simulink model "Nexonar_Navigation"  (R2018b)
settings: Solver=FixedStepDiscrete  StartTime=0.0  StopTime=0.1  RelTol=1e-3  EnableMultiTasking=on
libraries: commutil2 x12, c2833xlib x5, c280xlib x5, simulink x1, c2000lib x1
(part 2 of 2)

== stateflow chart Nexonar_Navigation/Nexonar-System/Navigationssystem [Einstellungen moeglich]/Fahrsystem ==
  state Fahren_mit_Ausrichtungsregelung
    entry:
    pwm_out_l = pwm_out - round(pwm_mindern(1) * (pwm_out / 100) ^ 2) * l_mindern;
    pwm_out_r = pwm_out - round(pwm_mindern(1) * (pwm_out / 100) ^ 2) * r_mindern;
    r_l_out_l = 1 - Gang;
    r_l_out_r = 1 - Gang;
  state Start_Warten
  state Drehen_links_max
    entry:
    pwm_out_l = 100;
    pwm_out_r = 100;
    r_l_out_l = 0;
    r_l_out_r = 1;
  state Drehen_rechts_max
    entry:
    pwm_out_l = 100;
    pwm_out_r = 100;
    r_l_out_l = 1;
    r_l_out_r = 0;
  state Drehen_links_gesteuert
    entry:
    pwm_out_l = 59 + abs(alpha_diff_opt);
    pwm_out_r = 59 + abs(alpha_diff_opt);
    r_l_out_l = 0;
    r_l_out_r = 1;
  state Drehen_rechts_gesteuert
    entry:
    pwm_out_l = 59 + abs(alpha_diff_opt);
    pwm_out_r = 59 + abs(alpha_diff_opt);
    r_l_out_l = 1;
    r_l_out_r = 0;
  (junction 81) -> Fahren_mit_Ausrichtungsregelung [order 1] : [pwm_mindern(2) == 1]
      | {l_mindern = 1 - Gang; r_mindern = 0 + Gang;}
  (junction 81) -> Fahren_mit_Ausrichtungsregelung [order 2] : [pwm_mindern(2) == 0]
      | {l_mindern = 0 + Gang; r_mindern = 1 - Gang;}
  (junction 1) -> (junction 81) [order 2]
  Fahren_mit_Ausrichtungsregelung -> (junction 32)
  (junction 81) -> Fahren_mit_Ausrichtungsregelung [order 3] : {l_mindern = 0; r_mindern = 0;}
  Start_Warten -> (junction 1)
  (junction 32) -> (junction 1)
  (default) -> Start_Warten
  Drehen_links_max -> (junction 32)
  Drehen_rechts_max -> (junction 32)
  Drehen_links_gesteuert -> (junction 32)
  (junction 1) -> (junction 18) [order 1] : [abs(alpha_diff_opt) > 0 && pwm_out > 0]
  Drehen_rechts_gesteuert -> (junction 32)
  (junction 18) -> (junction 44) [order 1] : [abs(alpha_diff_opt) > 40]
  (junction 44) -> Drehen_links_max [order 1] : [alpha_diff_opt > 0]
  (junction 18) -> (junction 52) [order 2]
  (junction 44) -> Drehen_rechts_max [order 2]
  (junction 52) -> Drehen_links_gesteuert [order 1] : [alpha_diff_opt > 0]
  (junction 52) -> Drehen_rechts_gesteuert [order 2]
  data: Gang input; pwm_out input; pwm_mindern input; alpha_diff_opt input; pwm_out_l output; pwm_out_r output; r_l_out_l output; r_l_out_r output; l_mindern local; r_mindern local

== stateflow chart Nexonar_Navigation/Nexonar-System/Navigationssystem [Einstellungen moeglich]/Drehweg-Optimierung mit Gang-Ausrichtung [Init: Stillstandintervall = ±15°] ==
  state Einstellung_Init
    entry:
    Stillstandintervall = 15;
    %%%
    pwm_mindern = [0 0];
  state Drehstillstand_mit_Ausrichtungsregelung
    entry:
    alpha_diff_opt = 0;
    if abs(alpha_diff_intern) < 5
    pwm_mindern(1) = round(abs(alpha_diff_intern));
    elseif abs(alpha_diff_intern) < 15
    pwm_mindern(1) = 5 + floor((abs(alpha_diff_intern) - 5) / 2);
    else
    pwm_mindern(1) = 10;
    end;
    if alpha_diff_intern < 0
    pwm_mindern(2) = 0;
    elseif alpha_diff_intern > 0
    pwm_mindern(2) = 1;
    else
    pwm_mindern(2) = 2;
    end;
  state Weiterleitung_bei_Drehzustand
    entry:
    alpha_diff_opt = alpha_diff_intern;
  (default) -> Einstellung_Init
  (junction 95) -> (junction 32)
  Einstellung_Init -> (junction 32)
  (junction 32) -> (junction 6) : {alpha_diff_intern = alpha_diff + 180 * Gang}
  (junction 6) -> (junction 68) [order 2]
  (junction 68) -> Drehstillstand_mit_Ausrichtungsregelung [order 1] : [abs(alpha_diff_intern) <= Stillstandintervall]
  Drehstillstand_mit_Ausrichtungsregelung -> (junction 95)
  (junction 6) -> (junction 13) [order 1] : [abs(alpha_diff_intern) > 180]
  (junction 13) -> (junction 68) [order 1] : [alpha_diff_intern > 0]
      | {alpha_diff_intern = -360 + alpha_diff_intern}
  Weiterleitung_bei_Drehzustand -> (junction 95)
  (junction 13) -> (junction 68) [order 2] : {alpha_diff_intern = 360 + alpha_diff_intern}
  (junction 68) -> Weiterleitung_bei_Drehzustand [order 2]
  data: pwm_mindern output; Gang input; alpha_diff input; alpha_diff_opt output; alpha_diff_intern local; Stillstandintervall local

== stateflow chart Nexonar_Navigation/Nexonar-System/Navigationssystem [Einstellungen moeglich]/Winkelregelungssystem (Soll-Ist-Abgleich & Ausrichtungsauswertung)/Quadrantenteiler ==
  state Quadrant_a
    entry:
    Quadrant = 0;
  state Quadrant_b
    entry:
    Quadrant = 1;
  state Start_Warten
  state Quadrant_c
    entry:
    Quadrant = 2;
  state Quadrant_d
    entry:
    Quadrant = 3;
  (junction 6) -> Quadrant_a [order 1] : [x_diff >= 0 && y_diff >= 0]
  Quadrant_a -> (junction 35)
  (junction 6) -> Quadrant_b [order 2] : [x_diff <= 0 && y_diff > 0]
  Quadrant_b -> (junction 35)
  Start_Warten -> (junction 6)
  (junction 35) -> (junction 6)
  (default) -> Start_Warten
  (junction 6) -> Quadrant_c [order 3] : [x_diff < 0 && y_diff <= 0]
  Quadrant_c -> (junction 35)
  (junction 6) -> Quadrant_d [order 4]
  Quadrant_d -> (junction 35)
  data: x_diff input; y_diff input; Quadrant output

== stateflow chart Nexonar_Navigation/Nexonar-System/Navigationssystem [Einstellungen moeglich]/Winkelregelungssystem (Soll-Ist-Abgleich & Ausrichtungsauswertung)/Winkelausgabe fuer Ausrichtung ==
  state Ausrichtung_ohne_Aenderung
    entry:
    alpha_neu = alpha_Wagen;
  state Start_Warten
  state Trigonometrische_Auswertung_in_Grad_fuer_Quadrant_1_3
    entry:
    alpha_neu = round(atan(abs(x_diff)/abs(y_diff))*360/(2*pi));
  state Trigonometrische_Auswertung_in_Grad_fuer_Quadrant_0_2
    entry:
    alpha_neu = round(atan(abs(y_diff)/abs(x_diff))*360/(2*pi));
  (junction 4) -> Ausrichtung_ohne_Aenderung [order 1] : [x_diff == 0 && y_diff == 0]
  Ausrichtung_ohne_Aenderung -> (junction 65)
  Start_Warten -> (junction 4)
  (junction 65) -> (junction 4)
  (default) -> Start_Warten
  (junction 4) -> Trigonometrische_Auswertung_in_Grad_fuer_Quadrant_1_3 [order 4]
  (junction 4) -> Trigonometrische_Auswertung_in_Grad_fuer_Quadrant_0_2 [order 2] : [x_diff > 0 && y_diff >= 0]
  Trigonometrische_Auswertung_in_Grad_fuer_Quadrant_0_2 -> (junction 65)
  (junction 4) -> Trigonometrische_Auswertung_in_Grad_fuer_Quadrant_0_2 [order 3] : [x_diff < 0 && y_diff <= 0]
  Trigonometrische_Auswertung_in_Grad_fuer_Quadrant_1_3 -> (junction 65)
  data: x_diff input; y_diff input; alpha_neu output; alpha_Wagen input

== stateflow chart Nexonar_Navigation/Nexonar-System/Nexonar-Positionsbestimmung/Chart2 ==
  state Daten_einlesen
  state x0
  state x1_1
    entry: int16y_bin[0] = int8y_1[0];
    int16y_bin[1] = int8y_1[1];
    int16y_bin[2] = int8y_1[2];
    int16y_bin[3] = int8y_1[3];
    int16y_bin[4] = int8y_1[4];
    int16y_bin[5] = int8y_1[5]
    int16y_bin[6] = int8y_1[6];
    int16y_bin[7] = int8y_1[7];
    int16y_bin[8] = int8y_2[0];
    int16y_bin[9] = int8y_2[1];
    int16y_bin[10] = int8y_2[2];
    int16y_bin[11] = int8y_2[3];
    int16y_bin[12] = int8y_2[4];
    int16y_bin[13] = int8y_2[5]
    int16y_bin[14] = int8y_2[6];
    int16y_bin[15] = int8y_2[7];
  x0 -> Daten_einlesen
  (default) -> x0
  Daten_einlesen -> x1_1
  x1_1 -> Daten_einlesen
  data: int8y_1 input size=8; int8y_2 input size=8; int16y_bin output size=16 =0

== stateflow chart Nexonar_Navigation/Nexonar-System/Nexonar-Positionsbestimmung/Chart4 ==
  state Daten_einlesen
  state x0
  state x1_1
    entry: int16a1_bin[0] = int8a1_1[0];
    int16a1_bin[1] = int8a1_1[1];
    int16a1_bin[2] = int8a1_1[2];
    int16a1_bin[3] = int8a1_1[3];
    int16a1_bin[4] = int8a1_1[4];
    int16a1_bin[5] = int8a1_1[5]
    int16a1_bin[6] = int8a1_1[6];
    int16a1_bin[7] = int8a1_1[7];
    int16a1_bin[8] = int8a1_2[0];
    int16a1_bin[9] = int8a1_2[1];
    int16a1_bin[10] = int8a1_2[2];
    int16a1_bin[11] = int8a1_2[3];
    int16a1_bin[12] = int8a1_2[4];
    int16a1_bin[13] = int8a1_2[5]
    int16a1_bin[14] = int8a1_2[6];
    int16a1_bin[15] = int8a1_2[7];
  x0 -> Daten_einlesen
  (default) -> x0
  Daten_einlesen -> x1_1
  x1_1 -> Daten_einlesen
  data: int8a1_1 input size=8; int8a1_2 input size=8; int16a1_bin output size=16 =0

== stateflow chart Nexonar_Navigation/Nexonar-System/Nexonar-Positionsbestimmung/Chart6 ==
  state Daten_einlesen
  state x0
  state x1_1
    entry: int16x_bin[0] = int8x_1[0];
    int16x_bin[1] = int8x_1[1];
    int16x_bin[2] = int8x_1[2];
    int16x_bin[3] = int8x_1[3];
    int16x_bin[4] = int8x_1[4];
    int16x_bin[5] = int8x_1[5]
    int16x_bin[6] = int8x_1[6];
    int16x_bin[7] = int8x_1[7];
    int16x_bin[8] = int8x_2[0];
    int16x_bin[9] = int8x_2[1];
    int16x_bin[10] = int8x_2[2];
    int16x_bin[11] = int8x_2[3];
    int16x_bin[12] = int8x_2[4];
    int16x_bin[13] = int8x_2[5]
    int16x_bin[14] = int8x_2[6];
    int16x_bin[15] = int8x_2[7];
  x0 -> Daten_einlesen
  (default) -> x0
  Daten_einlesen -> x1_1
  x1_1 -> Daten_einlesen
  data: int8x_1 input size=8; int8x_2 input size=8; int16x_bin output size=16 =0

== stateflow chart Nexonar_Navigation/Nexonar-System/Nexonar-Positionsbestimmung/Chart8 ==
  state wert_erkannt
    entry:
    values_out1[0] = in_data[0];
    values_out1[1] = in_data[1];
    values_out1[2] = in_data[2];
    values_out1[3] = in_data[3];
    values_out1[4] = in_data[4];
    values_out1[5] = in_data[5];
    values_out1[6] = in_data[6];
    values_out1[7] = in_data[7];
    values_out1[8] = in_data[8];
    values_out1[9] = in_data[9];
    values_out1[10] = in_data[10];
    values_out1[11] = in_data[11];
    values_out1[12] = in_data[12];
    values_out1[13] = in_data[13];
    values_out1[14] = in_data[14];
    values_out1[15] = in_data[15];
    values_out1[16] = in_data[16];
    values_out1[17] = in_data[17];
    values_out1[18] = in_data[18];
    values_out1[19] = in_data[19];
  state init
    entry: values_out1[0] = 0;
    values_out1[1] = 0;
    values_out1[2] = 0;
    values_out1[3] = 0;
    values_out1[4] = 0;
    values_out1[5] = 0;
    values_out1[6] = 0;
    values_out1[7] = 0;
    values_out1[8] = 0;
    values_out1[9] = 0;
    values_out1[10] = 0;
    values_out1[11] = 0;
    values_out1[12] = 0;
    values_out1[13] = 0;
    values_out1[14] = 0;
    values_out1[15] = 0;
    values_out1[16] = 0;
    values_out1[17] = 0;
    values_out1[18] = 0;
    values_out1[19] = 0;
  state Anfang_found_Schritt_uebertragen_weglassen_performance
    entry: x_found = x_found +1;
  state x5_valid_data_found1
    entry: valid_values1 = values_out1[search+1];
    valid_values2 = values_out1[search+2];
    valid_values3 = values_out1[search+3];
    valid_values4 = values_out1[search+4];
    valid_values5 = values_out1[search+5];
    valid_values6 = values_out1[search+6];
    valid_values7 = values_out1[search+7];
    valid_values8 = values_out1[search+8];
    zaehler = zaehler +1;
  state wert_erkannt2
    entry:
    search = 0;
    counter = counter + 1;
  state x1_search1
    entry: search = search + 1;
  x5_valid_data_found1 -> wert_erkannt
  (default) -> init
  x1_search1 -> wert_erkannt [order 3]
  init -> wert_erkannt
  Anfang_found_Schritt_uebertragen_weglassen_performance -> x5_valid_data_found1 [order 1] : [((values_out1[search]+values_out1[search+1]+values_out1[search+2]+values_out1[search+3]+values_out1[search+4]+values_out1[search+5]+values_out1[search+6]+values_out1[search+7]+values_out1[search+8])) == values_out1[search+9]]
  Anfang_found_Schritt_uebertragen_weglassen_performance -> x5_valid_data_found1 [order 2] : [((values_out1[search]+values_out1[search+1]+values_out1[search+2]+values_out1[search+3]+values_out1[search+4]+values_out1[search+5]+values_out1[search+6]+values_out1[search+7]+values_out1[search+8])-(256)) == values_out1[search+9]]
  wert_erkannt -> wert_erkannt2
  Anfang_found_Schritt_uebertragen_weglassen_performance -> x5_valid_data_found1 [order 3] : [((values_out1[search]+values_out1[search+1]+values_out1[search+2]+values_out1[search+3]+values_out1[search+4]+values_out1[search+5]+values_out1[search+6]+values_out1[search+7]+values_out1[search+8])-(512)) == values_out1[search+9]]
  Anfang_found_Schritt_uebertragen_weglassen_performance -> x5_valid_data_found1 [order 7] : [((values_out1[search]+values_out1[search+1]+values_out1[search+2]+values_out1[search+3]+values_out1[search+4]+values_out1[search+5]+values_out1[search+6]+values_out1[search+7]+values_out1[search+8])-(768)) == values_out1[search+9]]
  Anfang_found_Schritt_uebertragen_weglassen_performance -> x5_valid_data_found1 [order 6] : [((values_out1[search]+values_out1[search+1]+values_out1[search+2]+values_out1[search+3]+values_out1[search+4]+values_out1[search+5]+values_out1[search+6]+values_out1[search+7]+values_out1[search+8])-(1024)) == values_out1[search+9]]
  Anfang_found_Schritt_uebertragen_weglassen_performance -> x5_valid_data_found1 [order 5] : [((values_out1[search]+values_out1[search+1]+values_out1[search+2]+values_out1[search+3]+values_out1[search+4]+values_out1[search+5]+values_out1[search+6]+values_out1[search+7]+values_out1[search+8])-(1280)) == values_out1[search+9]]
  Anfang_found_Schritt_uebertragen_weglassen_performance -> x5_valid_data_found1 [order 4] : [((values_out1[search]+values_out1[search+1]+values_out1[search+2]+values_out1[search+3]+values_out1[search+4]+values_out1[search+5]+values_out1[search+6]+values_out1[search+7]+values_out1[search+8])-(1536)) == values_out1[search+9]]
  Anfang_found_Schritt_uebertragen_weglassen_performance -> x5_valid_data_found1 [order 8] : [((values_out1[search]+values_out1[search+1]+values_out1[search+2]+values_out1[search+3]+values_out1[search+4]+values_out1[search+5]+values_out1[search+6]+values_out1[search+7]+values_out1[search+8])-(1792)) == values_out1[search+9]]
  Anfang_found_Schritt_uebertragen_weglassen_performance -> x5_valid_data_found1 [order 10] : [((values_out1[search]+values_out1[search+1]+values_out1[search+2]+values_out1[search+3]+values_out1[search+4]+values_out1[search+5]+values_out1[search+6]+values_out1[search+7]+values_out1[search+8])-(2048)) == values_out1[search+9]]
  Anfang_found_Schritt_uebertragen_weglassen_performance -> x1_search1 [order 9]
  wert_erkannt2 -> Anfang_found_Schritt_uebertragen_weglassen_performance [order 1] : [values_out1[search] == 88]
  x1_search1 -> Anfang_found_Schritt_uebertragen_weglassen_performance [order 1] : [values_out1[search] == 88]
  wert_erkannt2 -> x1_search1 [order 2]
  x1_search1 -> x1_search1 [order 2] : [search < 19]
  data: in_data input size=20; values_out1 local int16 size=20; zaehler local int32 =0; search local int16; valid_values1 output int16 size=1; valid_values2 output int16 size=1; valid_values3 output int16 size=1; valid_values4 output int16 size=1; valid_values5 output int16 size=1; valid_values6 output int16 size=1; valid_values7 output int16 size=1; valid_values8 output int16 size=1; counter local int32 =0; x_found local int32 =0

== matlab function Nexonar_Navigation/Nexonar-System/Navigationssystem [Einstellungen moeglich]/Positionsregelungssystem (Soll-Ist-Abgleich & PWM-Auswertung)/Betrag pwm_x ==
  settings: updateMethod=DISCRETE  sampleTime=0.01
  data: x_diff_abs input; pwm_x output; Zielradius input
function pwm_x = fcn( x_diff_abs, Zielradius)

if Zielradius < x_diff_abs && x_diff_abs < 60 + Zielradius
    pwm_x = 60;
elseif x_diff_abs <= Zielradius
    pwm_x = 0;
elseif x_diff_abs >= 100 + Zielradius
    pwm_x = 100;
else
    pwm_x = x_diff_abs;
end

== matlab function Nexonar_Navigation/Nexonar-System/Navigationssystem [Einstellungen moeglich]/Positionsregelungssystem (Soll-Ist-Abgleich & PWM-Auswertung)/Betrag pwm_y ==
  settings: updateMethod=DISCRETE  sampleTime=0.01
  data: Zielradius input; y_diff_abs input; pwm_y output
function pwm_y = fcn(Zielradius, y_diff_abs)

if Zielradius < y_diff_abs && y_diff_abs < 60 + Zielradius
    pwm_y = 60;
elseif y_diff_abs <= Zielradius
    pwm_y = 0;
elseif y_diff_abs >= 100 + Zielradius
    pwm_y = 100;
else
    pwm_y = y_diff_abs;
end

== matlab function Nexonar_Navigation/Nexonar-System/Nexonar-Positionsbestimmung/I2C Reset (behebt Stabilitätsprobleme der I2C-Verbindung)/I2C Reset/I2C Reset ==
function fcn()
%#codegen

coder.ceval( 'reset_i2c' );

== matlab function Nexonar_Navigation/Nexonar-System/Nexonar-Positionsbestimmung/I2C Reset (behebt Stabilitätsprobleme der I2C-Verbindung)/I2C Reinitialisierung/I2C Reinitialisierung ==
function fcn()
%#codegen

coder.ceval( 'init_i2c' );
